simulink model "H8_6GDL_linealizar_pruebas"  (R2022b)
settings: Solver=VariableStepAuto  StartTime=0.0  StopTime=10.0  RelTol=1e-3
undefined symbols (not defined in the file or in its folder): ems, hems
settings Model: Creator=aceao  LastModifiedBy=aceao

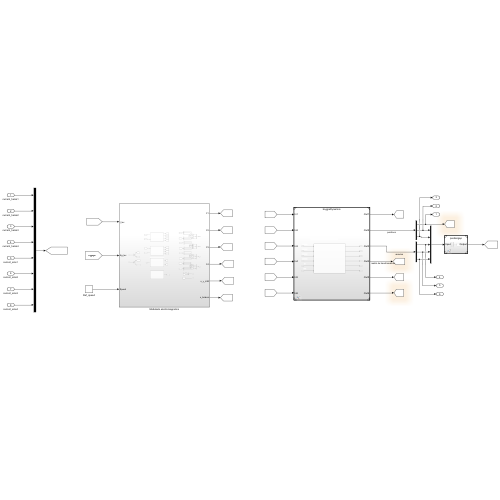
[thumbnail: Simulink's stored preview of the top-level diagram]
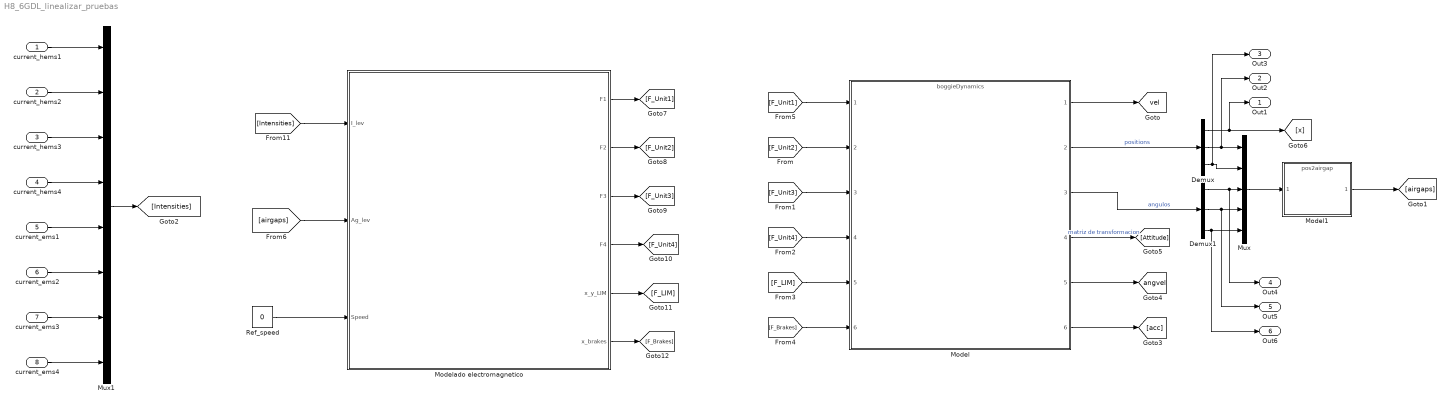
== system H8_6GDL_linealizar_pruebas ==
  current_hems1 : Inport
  current_hems2 : Inport  Port=2
  current_hems3 : Inport  Port=3
  current_hems4 : Inport  Port=4
  current_ems1 : Inport  Port=5
  current_ems2 : Inport  Port=6
  current_ems3 : Inport  Port=7
  current_ems4 : Inport  Port=8
  Demux : Demux  Outputs=3
  Demux1 : Demux  Outputs=3
  Model : ModelReference  ModelNameDialog=boggieDynamics.mdl  SimulationMode=Normal  ModelReferenceVersion=1.16
  Model1 : ModelReference  ModelNameDialog=pos2airgap.slx  SimulationMode=Normal  ModelReferenceVersion=1.2
  Modelado electromagnetico : Subsystem
  Mux : Mux  Inputs=5
  Mux1 : Mux  Inputs=8
  Ref_speed : Constant  Value=0
  Out1 : Outport
  Out2 : Outport  Port=2
  Out3 : Outport  Port=3
  Out4 : Outport  Port=4
  Out5 : Outport  Port=5
  Out6 : Outport  Port=6
  tag scope: angvel=global, vel=global
  wires:
  Model/4 -> [Attitude]  "matriz de transformacion"
  [F_Unit4] -> Model/4
  [F_LIM] -> Model/5
  Model1/1 -> [airgaps]
  Modelado electromagnetico/1(F1) -> [F_Unit1]
  [F_Brakes] -> Model/6
  Demux1/3 -> Out6/1, Mux/5
  Modelado electromagnetico/3(F3) -> [F_Unit3]
  Demux1/2 -> Out5/1, Mux/4
  [F_Unit2] -> Model/2
  [Intensities] -> Modelado electromagnetico/1(I_lev)
  [airgaps] -> Modelado electromagnetico/2(Ag_lev)
  Modelado electromagnetico/5(x_y_LIM) -> [F_LIM]
  Ref_speed/1 -> Modelado electromagnetico/3(Speed)
  Modelado electromagnetico/2(F2) -> [F_Unit2]
  Modelado electromagnetico/6(x_brakes) -> [F_Brakes]
  [F_Unit1] -> Model/1
  Demux1/1 -> Out4/1, Mux/3
  Modelado electromagnetico/4(F4) -> [F_Unit4]
  Mux/1 -> Model1/1
  Demux/2 -> Mux/1, Out2/1
  Model/1 -> [vel]
  Demux/1 -> Out1/1, [x]
  Model/2 -> Demux/1  "positions"
  [F_Unit3] -> Model/3
  Demux/3 -> Out3/1, Mux/2
  Model/6 -> [acc]
  Model/3 -> Demux1/1  "angulos"
  Model/5 -> [angvel]
  current_hems1/1 -> Mux1/1
  current_hems2/1 -> Mux1/2
  current_hems3/1 -> Mux1/3
  current_hems4/1 -> Mux1/4
  current_ems1/1 -> Mux1/5
  current_ems2/1 -> Mux1/6
  current_ems3/1 -> Mux1/7
  current_ems4/1 -> Mux1/8
  Mux1/1 -> [Intensities]

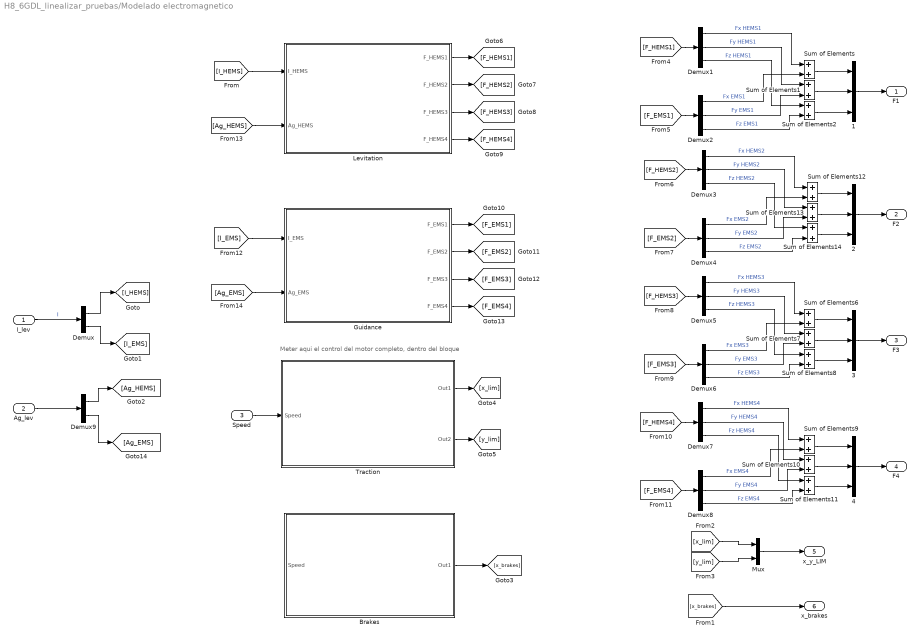
== system H8_6GDL_linealizar_pruebas/Modelado electromagnetico ==
  note: Meter aqui el control del motor completo, dentro del bloque
  I_lev : Inport
  Ag_lev : Inport  Port=2
  Speed : Inport  Port=3
  {1..4} (4 alike) : Mux  Inputs=3
  Brakes : Subsystem
  Demux : Demux  Outputs=2
  Demux{1..8} (8 alike) : Demux  Outputs=3
  Demux9 : Demux  Outputs=2
  Guidance : Subsystem
  Levitation : Subsystem
  Mux : Mux  Inputs=2
  Sum of Elements{,1..2,6..14} (12 alike) : Sum
  Traction : Subsystem
  F1 : Outport
  F2 : Outport  Port=2
  F3 : Outport  Port=3
  F4 : Outport  Port=4
  x_y_LIM : Outport  Port=5
  x_brakes : Outport  Port=6
  wires:
  I_lev/1 -> Demux/1  "I"
  Demux/1 -> [I_HEMS]
  Demux/2 -> [I_EMS]
  [I_HEMS] -> Levitation/1(I_HEMS)
  Brakes/1(Out1) -> [x_brakes]
  [x_brakes] -> x_brakes/1
  Traction/1(Out1) -> [x_lim]
  Traction/2(Out2) -> [y_lim]
  Mux/1 -> x_y_LIM/1
  [x_lim] -> Mux/1
  [y_lim] -> Mux/2
  Levitation/1(F_HEMS1) -> [F_HEMS1]
  Levitation/2(F_HEMS2) -> [F_HEMS2]
  Levitation/3(F_HEMS3) -> [F_HEMS3]
  Levitation/4(F_HEMS4) -> [F_HEMS4]
  Sum of Elements/1 -> 1/1
  1/1 -> F1/1
  Sum of Elements1/1 -> 1/2
  Sum of Elements2/1 -> 1/3
  2/1 -> F2/1
  [F_HEMS1] -> Demux1/1
  Demux1/1 -> Sum of Elements/1  "Fx HEMS1"
  Demux1/2 -> Sum of Elements1/1  "Fy HEMS1"
  Demux1/3 -> Sum of Elements2/1  "Fz HEMS1"
  3/1 -> F3/1
  Sum of Elements8/1 -> 3/3
  Sum of Elements6/1 -> 3/1
  Sum of Elements7/1 -> 3/2
  4/1 -> F4/1
  Sum of Elements11/1 -> 4/3
  Sum of Elements9/1 -> 4/1
  Sum of Elements10/1 -> 4/2
  Guidance/2(F_EMS2) -> [F_EMS2]
  Guidance/3(F_EMS3) -> [F_EMS3]
  Guidance/4(F_EMS4) -> [F_EMS4]
  Guidance/1(F_EMS1) -> [F_EMS1]
  Demux2/1 -> Sum of Elements/2  "Fx EMS1"
  [F_EMS1] -> Demux2/1
  Demux2/2 -> Sum of Elements1/2  "Fy EMS1"
  Demux2/3 -> Sum of Elements2/2  "Fz EMS1"
  [F_EMS2] -> Demux4/1
  Demux4/1 -> Sum of Elements12/2  "Fx EMS2"
  Demux4/2 -> Sum of Elements13/2  "Fy EMS2"
  Sum of Elements14/1 -> 2/3
  Demux3/1 -> Sum of Elements12/1  "Fx HEMS2"
  [F_HEMS2] -> Demux3/1
  Demux3/2 -> Sum of Elements13/1  "Fy HEMS2"
  Demux3/3 -> Sum of Elements14/1  "Fz HEMS2"
  Sum of Elements13/1 -> 2/2
  Sum of Elements12/1 -> 2/1
  Demux4/3 -> Sum of Elements14/2  "Fz EMS2"
  Demux5/3 -> Sum of Elements8/1  "Fz HEMS3"
  Demux5/2 -> Sum of Elements7/1  "Fy HEMS3"
  [F_HEMS3] -> Demux5/1
  Demux6/3 -> Sum of Elements8/2  "Fz EMS3"
  [F_EMS3] -> Demux6/1
  Demux6/1 -> Sum of Elements6/2  "Fx EMS3"
  Demux5/1 -> Sum of Elements6/1  "Fx HEMS3"
  Demux6/2 -> Sum of Elements7/2  "Fy EMS3"
  Demux7/3 -> Sum of Elements11/1  "Fz HEMS4"
  Demux8/3 -> Sum of Elements11/2  "Fz EMS4"
  Demux8/2 -> Sum of Elements10/2  "Fy EMS4"
  Demux7/2 -> Sum of Elements10/1  "Fy HEMS4"
  Demux7/1 -> Sum of Elements9/1  "Fx HEMS4"
  Demux8/1 -> Sum of Elements9/2  "Fx EMS4"
  [F_HEMS4] -> Demux7/1
  [F_EMS4] -> Demux8/1
  [I_EMS] -> Guidance/1(I_EMS)
  Ag_lev/1 -> Demux9/1
  Demux9/1 -> [Ag_HEMS]
  Demux9/2 -> [Ag_EMS]
  [Ag_HEMS] -> Levitation/2(Ag_HEMS)
  [Ag_EMS] -> Guidance/2(Ag_EMS)
  Speed/1 -> Traction/1(Speed)

== system H8_6GDL_linealizar_pruebas/Modelado electromagnetico/Brakes ==
  Speed : Inport
  2-D Lookup Table : Lookup_n-D  BreakpointsForDimension1=[1:3]  BreakpointsForDimension2=[1:3]  InternalRulePriority=Speed  RndMeth=Simplest
      settings: InputPortMap=u0,u1
  Out1 : Outport
  wires:
  Speed/1 -> 2-D Lookup Table/1

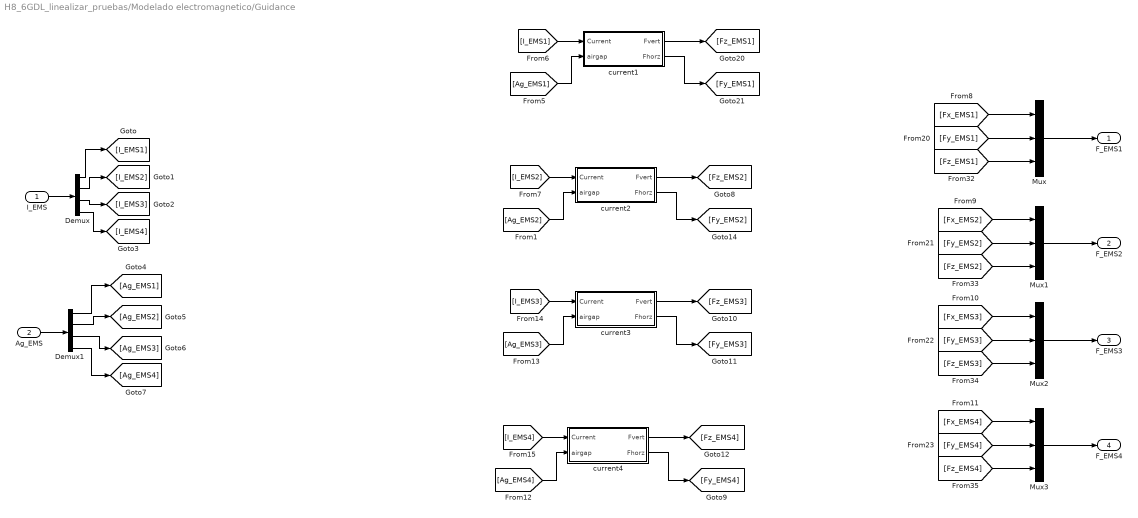
== system H8_6GDL_linealizar_pruebas/Modelado electromagnetico/Guidance ==
  I_EMS : Inport
  Ag_EMS : Inport  Port=2
  Demux : Demux
  Demux1 : Demux
  Mux{,1..3} (4 alike) : Mux  Inputs=3
  current1 : Subsystem
  current2 : Subsystem
  current3 : Subsystem
  current4 : Subsystem
  F_EMS1 : Outport
  F_EMS2 : Outport  Port=2
  F_EMS3 : Outport  Port=3
  F_EMS4 : Outport  Port=4
  wires:
  [Fz_EMS4] -> Mux3/3
  Demux1/4 -> [Ag_EMS4]
  [Fy_EMS1] -> Mux/2
  I_EMS/1 -> Demux/1
  Mux1/1 -> F_EMS2/1
  Demux/2 -> [I_EMS2]
  [Fy_EMS3] -> Mux2/2
  Mux3/1 -> F_EMS4/1
  [Fy_EMS4] -> Mux3/2
  [Fz_EMS1] -> Mux/3
  Mux/1 -> F_EMS1/1
  Mux2/1 -> F_EMS3/1
  [Fx_EMS3] -> Mux2/1
  Demux1/3 -> [Ag_EMS3]
  Ag_EMS/1 -> Demux1/1
  [Fz_EMS3] -> Mux2/3
  Demux/1 -> [I_EMS1]
  [Fz_EMS2] -> Mux1/3
  [Fx_EMS1] -> Mux/1
  Demux1/1 -> [Ag_EMS1]
  Demux/4 -> [I_EMS4]
  [Fx_EMS2] -> Mux1/1
  [Fy_EMS2] -> Mux1/2
  [Fx_EMS4] -> Mux3/1
  Demux/3 -> [I_EMS3]
  Demux1/2 -> [Ag_EMS2]
  current1/1(Fvert) -> [Fz_EMS1]
  current1/2(Fhorz) -> [Fy_EMS1]
  [Ag_EMS1] -> current1/2(airgap)
  [I_EMS1] -> current1/1(Current)
  current2/1(Fvert) -> [Fz_EMS2]
  [Ag_EMS2] -> current2/2(airgap)
  [I_EMS2] -> current2/1(Current)
  current2/2(Fhorz) -> [Fy_EMS2]
  current3/1(Fvert) -> [Fz_EMS3]
  [Ag_EMS3] -> current3/2(airgap)
  [Ag_EMS4] -> current4/2(airgap)
  current4/1(Fvert) -> [Fz_EMS4]
  [I_EMS3] -> current3/1(Current)
  [I_EMS4] -> current4/1(Current)
  current4/2(Fhorz) -> [Fy_EMS4]
  current3/2(Fhorz) -> [Fy_EMS3]

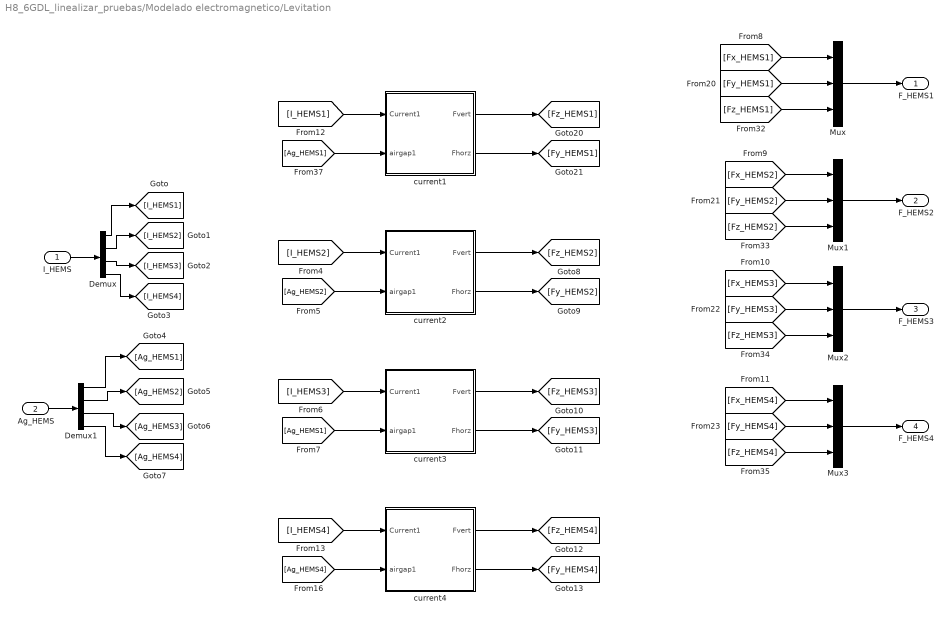
== system H8_6GDL_linealizar_pruebas/Modelado electromagnetico/Levitation ==
  I_HEMS : Inport
  Ag_HEMS : Inport  Port=2
  Demux : Demux
  Demux1 : Demux
  Mux{,1..3} (4 alike) : Mux  Inputs=3
  current1 : Subsystem
  current2 : Subsystem
  current3 : Subsystem
  current4 : Subsystem
  F_HEMS1 : Outport
  F_HEMS2 : Outport  Port=2
  F_HEMS3 : Outport  Port=3
  F_HEMS4 : Outport  Port=4
  wires:
  I_HEMS/1 -> Demux/1
  Mux/1 -> F_HEMS1/1
  Mux1/1 -> F_HEMS2/1
  Mux2/1 -> F_HEMS3/1
  Mux3/1 -> F_HEMS4/1
  Demux/1 -> [I_HEMS1]
  Demux/2 -> [I_HEMS2]
  Demux/3 -> [I_HEMS3]
  Demux/4 -> [I_HEMS4]
  Demux1/2 -> [Ag_HEMS2]
  Demux1/3 -> [Ag_HEMS3]
  Ag_HEMS/1 -> Demux1/1
  Demux1/4 -> [Ag_HEMS4]
  Demux1/1 -> [Ag_HEMS1]
  [Fx_HEMS1] -> Mux/1
  [Fx_HEMS2] -> Mux1/1
  [Fx_HEMS3] -> Mux2/1
  [Fx_HEMS4] -> Mux3/1
  [Fy_HEMS1] -> Mux/2
  [Fy_HEMS2] -> Mux1/2
  [Fy_HEMS3] -> Mux2/2
  [Fy_HEMS4] -> Mux3/2
  [Fz_HEMS1] -> Mux/3
  [Fz_HEMS2] -> Mux1/3
  [Fz_HEMS3] -> Mux2/3
  [Fz_HEMS4] -> Mux3/3
  current1/1(Fvert) -> [Fz_HEMS1]
  current1/2(Fhorz) -> [Fy_HEMS1]
  [I_HEMS1] -> current1/1(Current1)
  [Ag_HEMS1] -> current1/2(airgap1)
  current2/1(Fvert) -> [Fz_HEMS2]
  [Ag_HEMS2] -> current2/2(airgap1)
  current2/2(Fhorz) -> [Fy_HEMS2]
  [I_HEMS2] -> current2/1(Current1)
  current3/1(Fvert) -> [Fz_HEMS3]
  [Ag_HEMS1] -> current3/2(airgap1)
  [I_HEMS4] -> current4/1(Current1)
  [I_HEMS3] -> current3/1(Current1)
  current4/2(Fhorz) -> [Fy_HEMS4]
  current3/2(Fhorz) -> [Fy_HEMS3]
  current4/1(Fvert) -> [Fz_HEMS4]
  [Ag_HEMS4] -> current4/2(airgap1)

== system H8_6GDL_linealizar_pruebas/Modelado electromagnetico/Traction ==
  Speed : Inport
  Out1 : Outport
  Out2 : Outport  Port=2
  wires:
  Speed/1 -> Out1/1, Out2/1

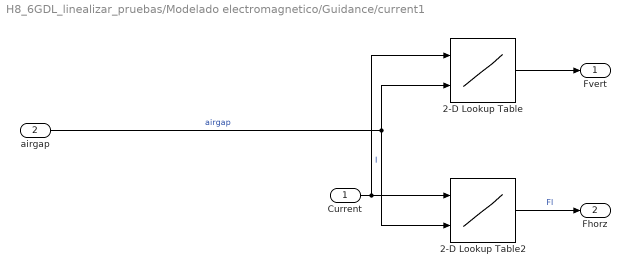
== system H8_6GDL_linealizar_pruebas/Modelado electromagnetico/Guidance/current1 ==
  Current : Inport
  airgap : Inport  Port=2
  2-D Lookup Table : Lookup_n-D  BreakpointsForDimension1=ems.Current  BreakpointsForDimension2=ems.Airgap'  Table=ems.Force_Vertical  InternalRulePriority=Speed  RndMeth=Simplest
      settings: InputPortMap=u0,u1
  2-D Lookup Table2 : Lookup_n-D  BreakpointsForDimension1=ems.Current  BreakpointsForDimension2=ems.Airgap'  Table=ems.Force_Horizontal  InternalRulePriority=Speed  RndMeth=Simplest
      settings: InputPortMap=u0,u1
  Fvert : Outport
  Fhorz : Outport  Port=2
  wires:
  2-D Lookup Table2/1 -> Fhorz/1  "Fl"
  Current/1 -> 2-D Lookup Table2/1, 2-D Lookup Table/1  "I"
  2-D Lookup Table/1 -> Fvert/1
  airgap/1 -> 2-D Lookup Table2/2, 2-D Lookup Table/2  "airgap"

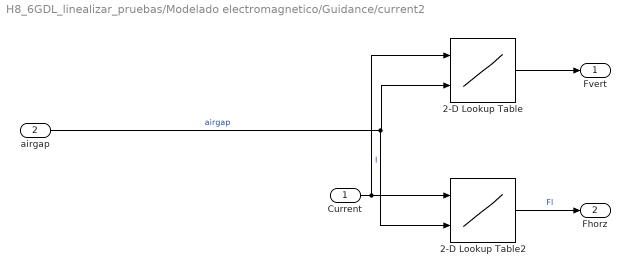
== system H8_6GDL_linealizar_pruebas/Modelado electromagnetico/Guidance/current2 ==
  Current : Inport
  airgap : Inport  Port=2
  2-D Lookup Table : Lookup_n-D  BreakpointsForDimension1=ems.Current  BreakpointsForDimension2=ems.Airgap'  Table=ems.Force_Vertical  InternalRulePriority=Speed  RndMeth=Simplest
      settings: InputPortMap=u0,u1
  2-D Lookup Table2 : Lookup_n-D  BreakpointsForDimension1=ems.Current  BreakpointsForDimension2=ems.Airgap'  Table=ems.Force_Horizontal  InternalRulePriority=Speed  RndMeth=Simplest
      settings: InputPortMap=u0,u1
  Fvert : Outport
  Fhorz : Outport  Port=2
  wires:
  2-D Lookup Table2/1 -> Fhorz/1  "Fl"
  Current/1 -> 2-D Lookup Table2/1, 2-D Lookup Table/1  "I"
  2-D Lookup Table/1 -> Fvert/1
  airgap/1 -> 2-D Lookup Table2/2, 2-D Lookup Table/2  "airgap"

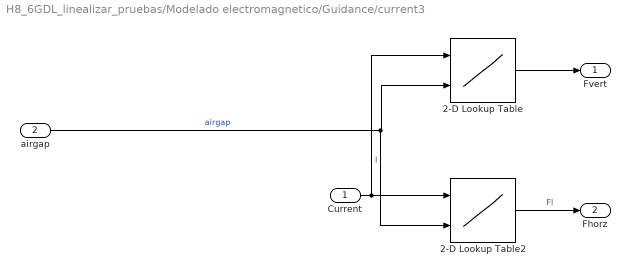
== system H8_6GDL_linealizar_pruebas/Modelado electromagnetico/Guidance/current3 ==
  Current : Inport
  airgap : Inport  Port=2
  2-D Lookup Table : Lookup_n-D  BreakpointsForDimension1=ems.Current  BreakpointsForDimension2=ems.Airgap'  Table=ems.Force_Vertical  InternalRulePriority=Speed  RndMeth=Simplest
      settings: InputPortMap=u0,u1
  2-D Lookup Table2 : Lookup_n-D  BreakpointsForDimension1=ems.Current  BreakpointsForDimension2=ems.Airgap'  Table=ems.Force_Horizontal  InternalRulePriority=Speed  RndMeth=Simplest
      settings: InputPortMap=u0,u1
  Fvert : Outport
  Fhorz : Outport  Port=2
  wires:
  2-D Lookup Table2/1 -> Fhorz/1  "Fl"
  Current/1 -> 2-D Lookup Table2/1, 2-D Lookup Table/1  "I"
  2-D Lookup Table/1 -> Fvert/1
  airgap/1 -> 2-D Lookup Table2/2, 2-D Lookup Table/2  "airgap"

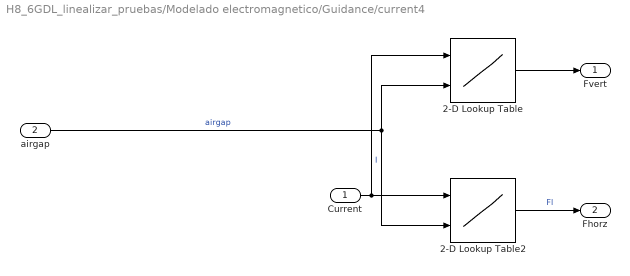
== system H8_6GDL_linealizar_pruebas/Modelado electromagnetico/Guidance/current4 ==
  Current : Inport
  airgap : Inport  Port=2
  2-D Lookup Table : Lookup_n-D  BreakpointsForDimension1=ems.Current  BreakpointsForDimension2=ems.Airgap'  Table=ems.Force_Vertical  InternalRulePriority=Speed  RndMeth=Simplest
      settings: InputPortMap=u0,u1
  2-D Lookup Table2 : Lookup_n-D  BreakpointsForDimension1=ems.Current  BreakpointsForDimension2=ems.Airgap'  Table=ems.Force_Horizontal  InternalRulePriority=Speed  RndMeth=Simplest
      settings: InputPortMap=u0,u1
  Fvert : Outport
  Fhorz : Outport  Port=2
  wires:
  2-D Lookup Table2/1 -> Fhorz/1  "Fl"
  Current/1 -> 2-D Lookup Table2/1, 2-D Lookup Table/1  "I"
  2-D Lookup Table/1 -> Fvert/1
  airgap/1 -> 2-D Lookup Table/2, 2-D Lookup Table2/2  "airgap"

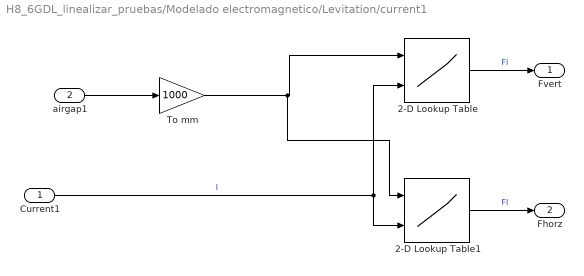
== system H8_6GDL_linealizar_pruebas/Modelado electromagnetico/Levitation/current1 ==
  Current1 : Inport
  airgap1 : Inport  Port=2
  2-D Lookup Table : Lookup_n-D  BreakpointsForDimension1=hems.Airgap'  BreakpointsForDimension2=hems.Current  Table=hems.Force_Vertical  InternalRulePriority=Speed  RndMeth=Simplest
      settings: InputPortMap=u0,u1
  2-D Lookup Table1 : Lookup_n-D  BreakpointsForDimension1=hems.Airgap'  BreakpointsForDimension2=hems.Current  Table=hems.Force_Horizontal  InternalRulePriority=Speed  RndMeth=Simplest
      settings: InputPortMap=u0,u1
  To mm : Gain  Gain=1000
  Fvert : Outport
  Fhorz : Outport  Port=2
  wires:
  2-D Lookup Table1/1 -> Fhorz/1  "Fl"
  2-D Lookup Table/1 -> Fvert/1  "Fl"
  Current1/1 -> 2-D Lookup Table1/2, 2-D Lookup Table/2  "I"
  airgap1/1 -> To mm/1
  To mm/1 -> 2-D Lookup Table1/1, 2-D Lookup Table/1

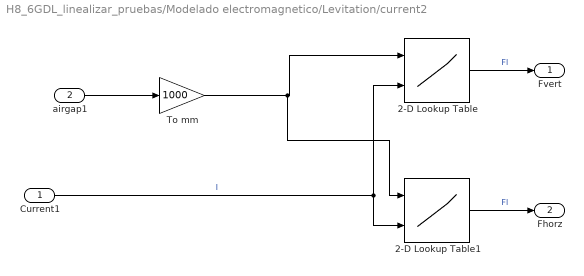
== system H8_6GDL_linealizar_pruebas/Modelado electromagnetico/Levitation/current2 ==
  Current1 : Inport
  airgap1 : Inport  Port=2
  2-D Lookup Table : Lookup_n-D  BreakpointsForDimension1=hems.Airgap'  BreakpointsForDimension2=hems.Current  Table=hems.Force_Vertical  InternalRulePriority=Speed  RndMeth=Simplest
      settings: InputPortMap=u0,u1
  2-D Lookup Table1 : Lookup_n-D  BreakpointsForDimension1=hems.Airgap'  BreakpointsForDimension2=hems.Current  Table=hems.Force_Horizontal  InternalRulePriority=Speed  RndMeth=Simplest
      settings: InputPortMap=u0,u1
  To mm : Gain  Gain=1000
  Fvert : Outport
  Fhorz : Outport  Port=2
  wires:
  2-D Lookup Table1/1 -> Fhorz/1  "Fl"
  2-D Lookup Table/1 -> Fvert/1  "Fl"
  Current1/1 -> 2-D Lookup Table1/2, 2-D Lookup Table/2  "I"
  airgap1/1 -> To mm/1
  To mm/1 -> 2-D Lookup Table1/1, 2-D Lookup Table/1

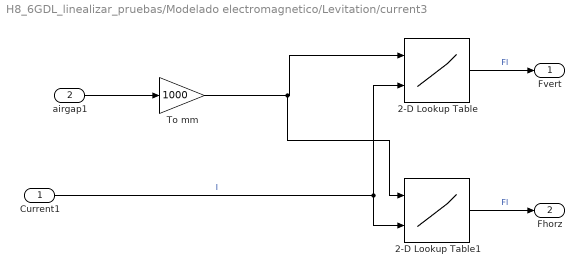
== system H8_6GDL_linealizar_pruebas/Modelado electromagnetico/Levitation/current3 ==
  Current1 : Inport
  airgap1 : Inport  Port=2
  2-D Lookup Table : Lookup_n-D  BreakpointsForDimension1=hems.Airgap'  BreakpointsForDimension2=hems.Current  Table=hems.Force_Vertical  InternalRulePriority=Speed  RndMeth=Simplest
      settings: InputPortMap=u0,u1
  2-D Lookup Table1 : Lookup_n-D  BreakpointsForDimension1=hems.Airgap'  BreakpointsForDimension2=hems.Current  Table=hems.Force_Horizontal  InternalRulePriority=Speed  RndMeth=Simplest
      settings: InputPortMap=u0,u1
  To mm : Gain  Gain=1000
  Fvert : Outport
  Fhorz : Outport  Port=2
  wires:
  2-D Lookup Table1/1 -> Fhorz/1  "Fl"
  2-D Lookup Table/1 -> Fvert/1  "Fl"
  Current1/1 -> 2-D Lookup Table1/2, 2-D Lookup Table/2  "I"
  airgap1/1 -> To mm/1
  To mm/1 -> 2-D Lookup Table1/1, 2-D Lookup Table/1

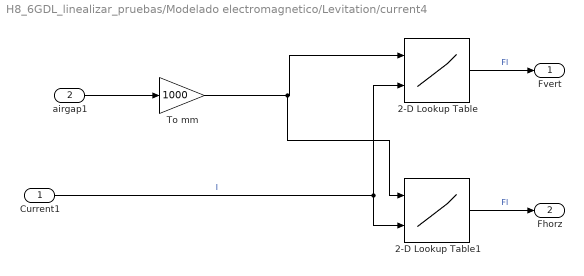
== system H8_6GDL_linealizar_pruebas/Modelado electromagnetico/Levitation/current4 ==
  Current1 : Inport
  airgap1 : Inport  Port=2
  2-D Lookup Table : Lookup_n-D  BreakpointsForDimension1=hems.Airgap'  BreakpointsForDimension2=hems.Current  Table=hems.Force_Vertical  InternalRulePriority=Speed  RndMeth=Simplest
      settings: InputPortMap=u0,u1
  2-D Lookup Table1 : Lookup_n-D  BreakpointsForDimension1=hems.Airgap'  BreakpointsForDimension2=hems.Current  Table=hems.Force_Horizontal  InternalRulePriority=Speed  RndMeth=Simplest
      settings: InputPortMap=u0,u1
  To mm : Gain  Gain=1000
  Fvert : Outport
  Fhorz : Outport  Port=2
  wires:
  2-D Lookup Table1/1 -> Fhorz/1  "Fl"
  2-D Lookup Table/1 -> Fvert/1  "Fl"
  Current1/1 -> 2-D Lookup Table1/2, 2-D Lookup Table/2  "I"
  airgap1/1 -> To mm/1
  To mm/1 -> 2-D Lookup Table1/1, 2-D Lookup Table/1
